simulink model "Luenberger_Non_Linear"  (R2017b)
settings: Solver=VariableStepAuto  StartTime=0.0  StopTime=100  RelTol=1e-3
values from neighbouring files (symbols this model uses):
  A = [0,1,0,0,0,0;0,0,-m1*g/M,0,-m2*g/M,0;0,0,0,1,0,0;0,0,-(M+m1)*g/(M*l1),0,-m2*g/(M*l1),0;0,0,0,0,0,1;0,0,-(m1)*g/(M*l2),0,-(m2+M)*g/(M*l2),0]    [Controls_project.m]
  B = [0;1/M;0;1/(M*l1);0;1/(M*l2)]    [Controls_project.m]
  C = [1,0,0,0,0,0;0,0,1,0,0,0;0,0,0,0,1,0]    [Controls_project.m]
  C1 = [1 0 0 0 0 0; 0 0 0 0 0 0; 0 0 0 0 0 0]    [Controls_project.m]
  D = [0;0;0]    [Controls_project.m]
  g = 9.8    [Controls_project.m]
  K = lqr(A,B,q,r)    [Controls_project.m]
  l1 = 20    [Controls_project.m]
  l2 = 10    [Controls_project.m]
  M = 1000    [Controls_project.m]
  m1 = 100    [Controls_project.m]
  m2 = 100    [Controls_project.m]
libraries: peLuenbergerObserver x1
settings Model: Creator=Adheesh  LastModifiedBy=Adheesh

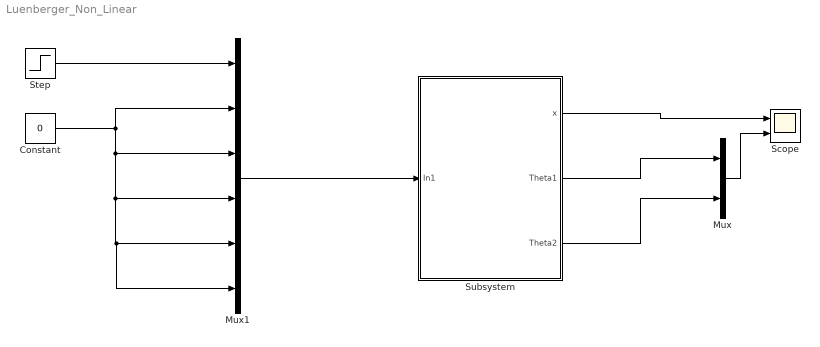
== system Luenberger_Non_Linear ==
  Constant : Constant  Value=0
  Mux : Mux  Inputs=2
  Mux1 : Mux  Inputs=6
  Scope : Scope  NumInputPorts=2
  Step : Step  Time=5  SampleTime=0
  Subsystem : Subsystem
  wires:
  Constant/1 -> Mux1/6, Mux1/5, Mux1/4, Mux1/3, Mux1/2
  Step/1 -> Mux1/1
  Mux/1 -> Scope/2
  Subsystem/1("x ") -> Scope/1
  Subsystem/2(Theta1) -> Mux/1
  Subsystem/3(Theta2) -> Mux/2
  Mux1/1 -> Subsystem/1(In1)

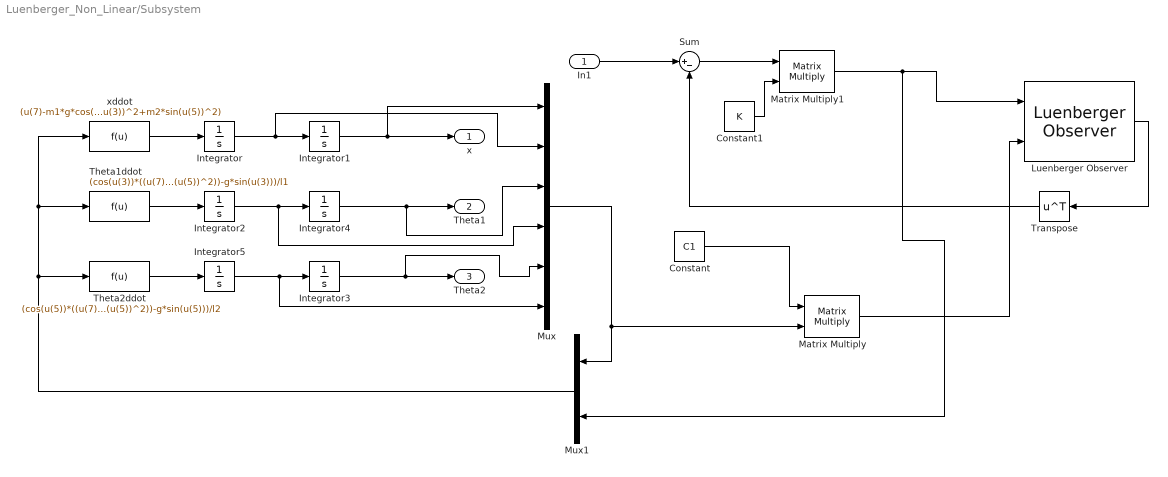
== system Luenberger_Non_Linear/Subsystem ==
  In1 : Inport
  Constant : Constant  Value=C1
  Constant1 : Constant  Value=K
  Integrator{,1..5} (6 alike) : Integrator
  Luenberger Observer : peLuenbergerObserver/Luenberger Observer  StateSpaceType=Continuous-time  Ad=A  Bd=B  Cd=C  Dd=D  A=A  B=B  C=C  D=D  ObserverDesign=Desired eigenvalues  Ld=1  DesiredEigenvalues=obsr_poles  x0=[0;0;0;0;0;0]  Tsd=0.1  Ts=0.1
  Matrix Multiply : Product  Multiplication=Matrix(*)
  Matrix Multiply1 : Product  Multiplication=Matrix(*)
  Mux : Mux  Inputs=6
  Mux1 : Mux  Inputs=2
  Sum : Sum  Inputs=|+-
  Theta1ddot : Fcn  Expr=(cos(u(3))*((u(7)-m1*g*cos(u(3))*sin(u(3))-m2*g*cos(u(5))*sin(u(5))-m1*l1*sin(u(3))*u(4)^2-m2*l2*sin(u(5))*u(6)^2)/(M+m1*sin(u(3))^2+m2*sin(u(5))^2))-g*sin(u(3)))/l1
  "Theta2ddot " : Fcn  Expr=(cos(u(5))*((u(7)-m1*g*cos(u(3))*sin(u(3))-m2*g*cos(u(5))*sin(u(5))-m1*l1*sin(u(3))*u(4)^2-m2*l2*sin(u(5))*u(6)^2)/(M+m1*sin(u(3))^2+m2*sin(u(5))^2))-g*sin(u(5)))/l2
  Transpose : Math  Operator=transpose  SaturateOnIntegerOverflow=on
  "xddot " : Fcn  Expr=(u(7)-m1*g*cos(u(3))*sin(u(3))-m2*g*cos(u(5))*sin(u(5))-m1*l1*sin(u(3))*u(4)^2-m2*l2*sin(u(5))*u(6)^2)/(M+m1*sin(u(3))^2+m2*sin(u(5))^2)
  "x " : Outport
  Theta1 : Outport  Port=2
  Theta2 : Outport  Port=3
  wires:
  In1/1 -> Sum/1
  Sum/1 -> Matrix Multiply1/1
  Constant1/1 -> Matrix Multiply1/2
  Matrix Multiply1/1 -> Mux1/2, Luenberger Observer/1
  Mux/1 -> Mux1/1, Matrix Multiply/2
  Constant/1 -> Matrix Multiply/1
  Matrix Multiply/1 -> Luenberger Observer/2
  "Theta2ddot "/1 -> Integrator5/1
  Integrator5/1 -> Mux/6, Integrator3/1
  Mux1/1 -> "Theta2ddot "/1, Theta1ddot/1, "xddot "/1
  Integrator2/1 -> Mux/4, Integrator4/1
  Integrator3/1 -> Theta2/1, Mux/5
  Integrator1/1 -> "x "/1, Mux/1
  Integrator/1 -> Mux/2, Integrator1/1
  Integrator4/1 -> Theta1/1, Mux/3
  Theta1ddot/1 -> Integrator2/1
  "xddot "/1 -> Integrator/1
  Luenberger Observer/1 -> Transpose/1
  Transpose/1 -> Sum/2
